simulink model "Model_statespacesystem"  (R2024b)
settings: Solver=ode45  StartTime=0.0  StopTime=30  RelTol=1e-3
settings Model: Creator=Riccardo Grosso  LastModifiedBy=Buton
settings DataIOCC: ReturnWorkspaceOutputs=off

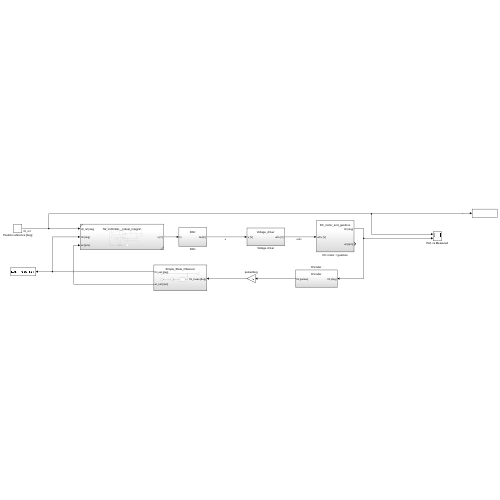
[thumbnail: Simulink's stored preview of the top-level diagram]
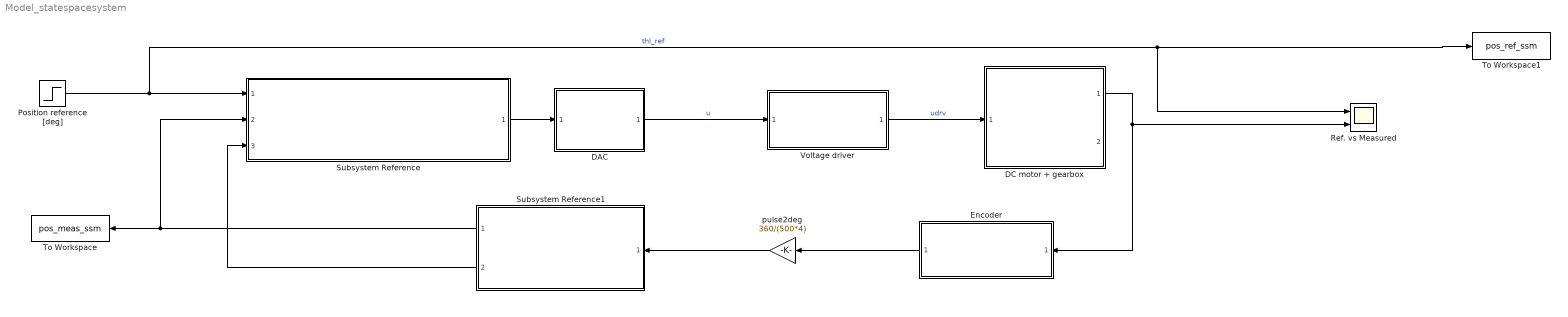
== system Model_statespacesystem ==
  DAC : Subsystem  ReferencedSubsystem=DAC
  DC motor + gearbox : Subsystem  ReferencedSubsystem=DC_motor_and_gearbox
  Encoder : Subsystem  ReferencedSubsystem=Encoder
  Position reference [deg] : Step  Time=0  After=120  SampleTime=0
  Ref. vs Measured : Scope  NumInputPorts=2
  Subsystem Reference : Subsystem  ReferencedSubsystem=Ss_controller__robust_integral
  Subsystem Reference1 : Subsystem  ReferencedSubsystem=Simple_State_Observer
  To Workspace : ToWorkspace  VariableName=pos_meas_ssm  SaveFormat=Timeseries  SampleTime=-1
  To Workspace1 : ToWorkspace  VariableName=pos_ref_ssm  SaveFormat=Timeseries  SampleTime=-1
  Voltage driver : Subsystem  ReferencedSubsystem=Voltage_driver
  pulse2deg : Gain  Gain=360/(500*4)
  wires:
  DAC/1 -> Voltage driver/1  "u"
  Voltage driver/1 -> DC motor + gearbox/1  "udrv"
  Encoder/1 -> pulse2deg/1
  DC motor + gearbox/1 -> Encoder/1, Ref. vs Measured/2
  Position reference [deg]/1 -> Subsystem Reference/1, To Workspace1/1, Ref. vs Measured/1  "thl_ref"
  Subsystem Reference/1 -> DAC/1
  pulse2deg/1 -> Subsystem Reference1/1
  Subsystem Reference1/1 -> Subsystem Reference/2, To Workspace/1
  Subsystem Reference1/2 -> Subsystem Reference/3
